simulink model "PMSM_Control"  (R2024b)
settings: Solver=VariableStepAuto  StartTime=0.0  StopTime=0.1  MaxStep=1e-3  RelTol=1e-3
values from neighbouring files (symbols this model uses):
  Ipeak = 2    [PMSM_Data.m]
  Ls = 0.01    [PMSM_Data.m]
  R = 1    [PMSM_Data.m]
  Vpeak = 12    [PMSM_Data.m]
  w = 300    [PMSM_Data.m]
libraries: mcbcontrolslib x1
settings Model: Creator=MOHAMED  LastModifiedBy=MOHAMED

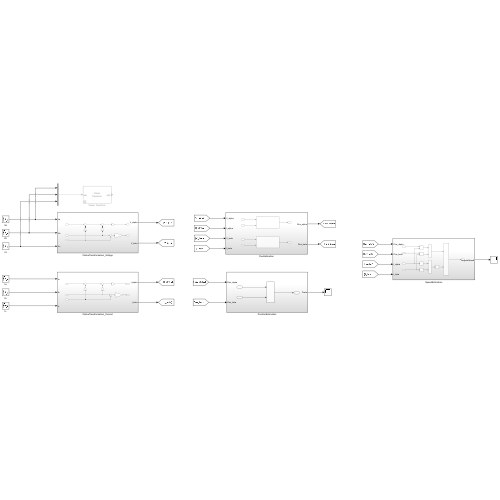
[thumbnail: Simulink's stored preview of the top-level diagram]
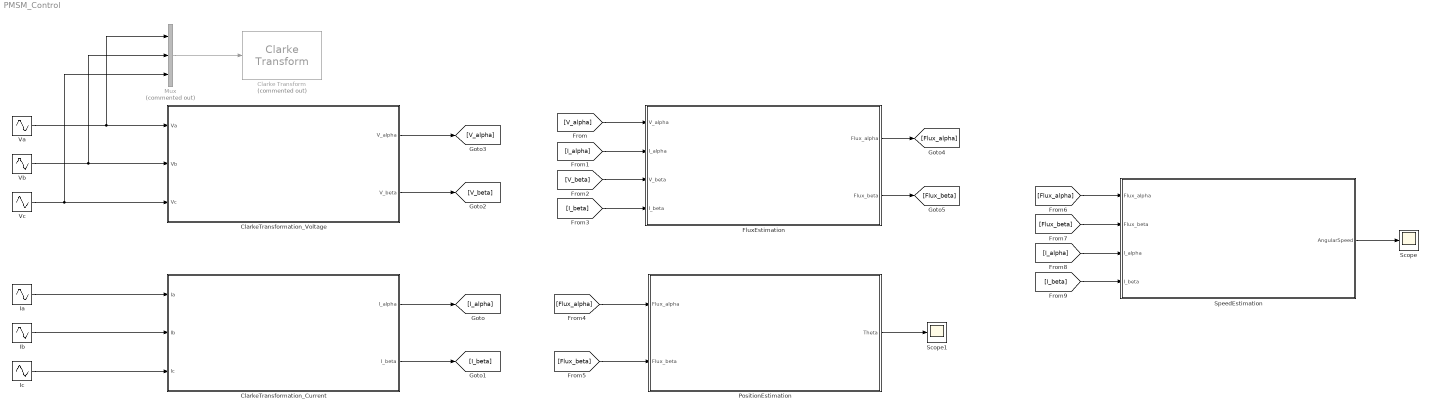
== system PMSM_Control ==
  Clarke Transform : mcbcontrolslib/Clarke Transform  Commented=on  VariantControl=Variant2  PhaseInput=Three inputs  EnPowerInv=off
      settings: LibrarySourceBlock=mcblib/Controls/Math Transforms/Clarke Transform
  ClarkeTransformation_Current : Subsystem
  ClarkeTransformation_Voltage : Subsystem
  FluxEstimation : Subsystem
  Ia : Sin  Amplitude=Ipeak  Frequency=w  Phase=deg2rad(0)  SampleTime=0
  Ib : Sin  Amplitude=Ipeak  Frequency=w  Phase=deg2rad(120)  SampleTime=0
  Ic : Sin  Amplitude=Ipeak  Frequency=w  Phase=deg2rad(-120)  SampleTime=0
  Mux : Mux  Commented=on  Inputs=3
  PositionEstimation : Subsystem
  Scope : Scope
  Scope1 : Scope
  SpeedEstimation : Subsystem
  Va : Sin  Amplitude=Vpeak  Frequency=w  Phase=deg2rad(0)  SampleTime=0
  Vb : Sin  Amplitude=Vpeak  Frequency=w  Phase=deg2rad(120)  SampleTime=0
  Vc : Sin  Amplitude=Vpeak  Frequency=w  Phase=deg2rad(-120)  SampleTime=0
  wires:
  Vc/1 -> Mux/3, ClarkeTransformation_Voltage/3(Vc)
  Vb/1 -> Mux/2, ClarkeTransformation_Voltage/2(Vb)
  Va/1 -> Mux/1, ClarkeTransformation_Voltage/1(Va)
  Mux/1 -> Clarke Transform/1
  Ic/1 -> ClarkeTransformation_Current/3(Ic)
  Ib/1 -> ClarkeTransformation_Current/2(Ib)
  Ia/1 -> ClarkeTransformation_Current/1(Ia)
  ClarkeTransformation_Current/1(I_alpha) -> [I_alpha]
  ClarkeTransformation_Current/2(I_beta) -> [I_beta]
  ClarkeTransformation_Voltage/2(V_beta) -> [V_beta]
  ClarkeTransformation_Voltage/1(V_alpha) -> [V_alpha]
  [V_alpha] -> FluxEstimation/1(V_alpha)
  [I_alpha] -> FluxEstimation/2(I_alpha)
  [V_beta] -> FluxEstimation/3(V_beta)
  [I_beta] -> FluxEstimation/4(I_beta)
  FluxEstimation/1(Flux_alpha) -> [Flux_alpha]
  FluxEstimation/2(Flux_beta) -> [Flux_beta]
  [Flux_alpha] -> PositionEstimation/1(Flux_alpha)
  [Flux_beta] -> PositionEstimation/2(Flux_beta)
  PositionEstimation/1(Theta) -> Scope1/1
  [Flux_alpha] -> SpeedEstimation/1(Flux_alpha)
  [Flux_beta] -> SpeedEstimation/2(Flux_beta)
  [I_alpha] -> SpeedEstimation/3(I_alpha)
  [I_beta] -> SpeedEstimation/4(I_beta)
  SpeedEstimation/1(AngularSpeed) -> Scope/1

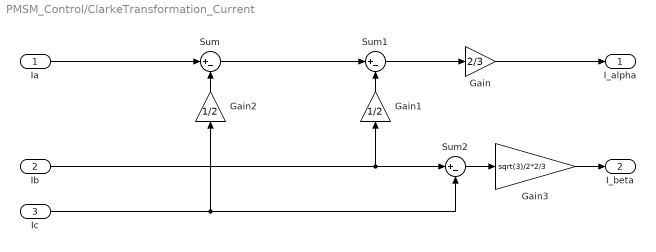
== system PMSM_Control/ClarkeTransformation_Current ==
  Ia : Inport
  Ib : Inport  Port=2
  Ic : Inport  Port=3
  Gain : Gain  Gain=2/3
  Gain1 : Gain  Gain=1/2
  Gain2 : Gain  Gain=1/2
  Gain3 : Gain  Gain=sqrt(3)/2*2/3
  Sum : Sum  Inputs=|+-
  Sum1 : Sum  Inputs=|+-
  Sum2 : Sum  Inputs=|+-
  I_alpha : Outport
  I_beta : Outport  Port=2
  wires:
  Gain3/1 -> I_beta/1
  Sum2/1 -> Gain3/1
  Gain1/1 -> Sum1/2
  Gain2/1 -> Sum/2
  Ib/1 -> Sum2/1, Gain1/1
  Ic/1 -> Gain2/1, Sum2/2
  Gain/1 -> I_alpha/1
  Sum1/1 -> Gain/1
  Sum/1 -> Sum1/1
  Ia/1 -> Sum/1

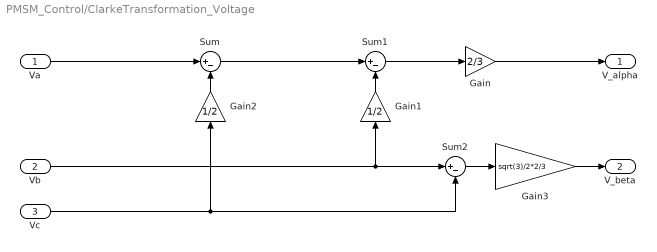
== system PMSM_Control/ClarkeTransformation_Voltage ==
  Va : Inport
  Vb : Inport  Port=2
  Vc : Inport  Port=3
  Gain : Gain  Gain=2/3
  Gain1 : Gain  Gain=1/2
  Gain2 : Gain  Gain=1/2
  Gain3 : Gain  Gain=sqrt(3)/2*2/3
  Sum : Sum  Inputs=|+-
  Sum1 : Sum  Inputs=|+-
  Sum2 : Sum  Inputs=|+-
  V_alpha : Outport
  V_beta : Outport  Port=2
  wires:
  Va/1 -> Sum/1
  Sum/1 -> Sum1/1
  Sum1/1 -> Gain/1
  Gain/1 -> V_alpha/1
  Vc/1 -> Sum2/2, Gain2/1
  Vb/1 -> Gain1/1, Sum2/1
  Gain2/1 -> Sum/2
  Gain1/1 -> Sum1/2
  Sum2/1 -> Gain3/1
  Gain3/1 -> V_beta/1

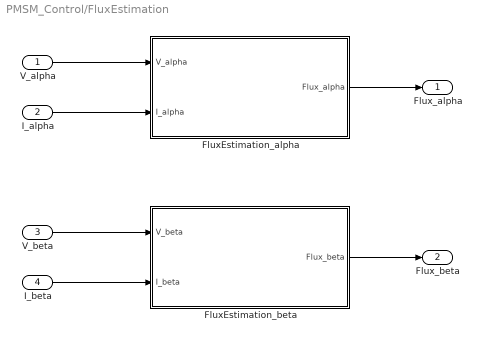
== system PMSM_Control/FluxEstimation ==
  V_alpha : Inport
  I_alpha : Inport  Port=2
  V_beta : Inport  Port=3
  I_beta : Inport  Port=4
  FluxEstimation_alpha : Subsystem
  FluxEstimation_beta : Subsystem
  Flux_alpha : Outport
  Flux_beta : Outport  Port=2
  wires:
  V_alpha/1 -> FluxEstimation_alpha/1(V_alpha)
  I_alpha/1 -> FluxEstimation_alpha/2(I_alpha)
  FluxEstimation_alpha/1(Flux_alpha) -> Flux_alpha/1
  FluxEstimation_beta/1(Flux_beta) -> Flux_beta/1
  V_beta/1 -> FluxEstimation_beta/1(V_beta)
  I_beta/1 -> FluxEstimation_beta/2(I_beta)

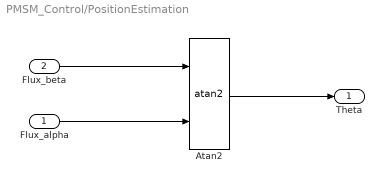
== system PMSM_Control/PositionEstimation ==
  Flux_alpha : Inport
  Flux_beta : Inport  Port=2
  Atan2 : Trigonometry  Operator=atan2
  Theta : Outport
  wires:
  Atan2/1 -> Theta/1
  Flux_beta/1 -> Atan2/1
  Flux_alpha/1 -> Atan2/2

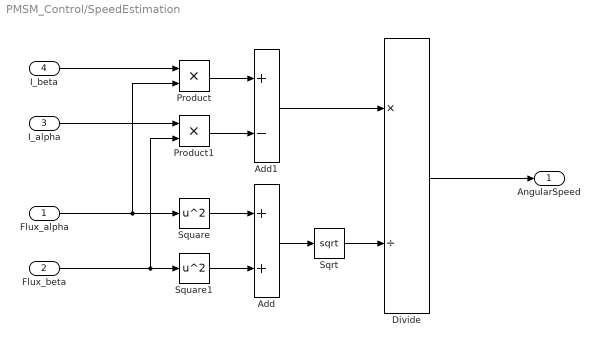
== system PMSM_Control/SpeedEstimation ==
  Flux_alpha : Inport
  Flux_beta : Inport  Port=2
  I_alpha : Inport  Port=3
  I_beta : Inport  Port=4
  Add : Sum
  Add1 : Sum  Inputs=+-
  Divide : Product  Inputs=*/
  Product : Product
  Product1 : Product
  Sqrt : Sqrt
  Square : Math  Operator=square
  Square1 : Math  Operator=square
  AngularSpeed : Outport
  wires:
  Square1/1 -> Add/2
  Square/1 -> Add/1
  Product/1 -> Add1/1
  Product1/1 -> Add1/2
  Add1/1 -> Divide/1
  Add/1 -> Sqrt/1
  Divide/1 -> AngularSpeed/1
  Sqrt/1 -> Divide/2
  Flux_alpha/1 -> Product/2, Square/1
  Flux_beta/1 -> Product1/2, Square1/1
  I_beta/1 -> Product/1
  I_alpha/1 -> Product1/1

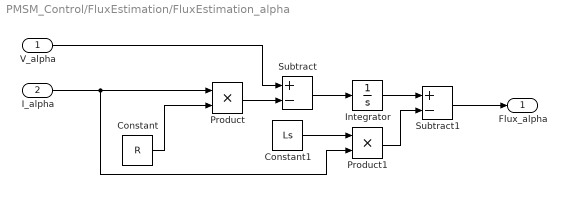
== system PMSM_Control/FluxEstimation/FluxEstimation_alpha ==
  V_alpha : Inport
  I_alpha : Inport  Port=2
  Constant : Constant  Value=R
  Constant1 : Constant  Value=Ls
  Integrator : Integrator
  Product : Product
  Product1 : Product
  Subtract : Sum  Inputs=+-
  Subtract1 : Sum  Inputs=+-
  Flux_alpha : Outport
  wires:
  Product1/1 -> Subtract1/2
  V_alpha/1 -> Subtract/1
  Product/1 -> Subtract/2
  Constant/1 -> Product/2
  Constant1/1 -> Product1/1
  Integrator/1 -> Subtract1/1
  Subtract/1 -> Integrator/1
  Subtract1/1 -> Flux_alpha/1
  I_alpha/1 -> Product/1, Product1/2

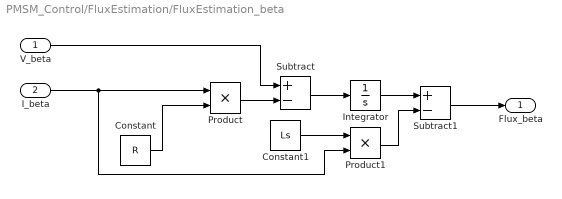
== system PMSM_Control/FluxEstimation/FluxEstimation_beta ==
  V_beta : Inport
  I_beta : Inport  Port=2
  Constant : Constant  Value=R
  Constant1 : Constant  Value=Ls
  Integrator : Integrator
  Product : Product
  Product1 : Product
  Subtract : Sum  Inputs=+-
  Subtract1 : Sum  Inputs=+-
  Flux_beta : Outport
  wires:
  I_beta/1 -> Product1/2, Product/1
  Subtract1/1 -> Flux_beta/1
  Subtract/1 -> Integrator/1
  Integrator/1 -> Subtract1/1
  Constant1/1 -> Product1/1
  Constant/1 -> Product/2
  Product/1 -> Subtract/2
  V_beta/1 -> Subtract/1
  Product1/1 -> Subtract1/2
